simulink model "lab5_extra"  (R2017b)
settings: Solver=FixedStepDiscrete  StartTime=0.0  StopTime=5  RelTol=1e-3
InitFcn:
  | load speech_signal;
  | Fs = 8000;
  | Ts = 1/Fs;
  | 
  | DPRAM1_size = 2048; %number of words
  | DPRAM1_address_size = log2(DPRAM1_size);
  | 
  | FFT_size = 1024;
  | FFT_size_half = FFT_size;
  | FFT_frame_shift = 256;
  | FFT_frame_shift_Nbits = log2(FFT_frame_shift);
  | 
  | SysRate_Upsample_Factor = 32;
libraries: hdlsllib x16, simulink x5, dspxfrm3 x2, dspsigops x1
settings Model: Creator=Ross_admin  LastModifiedBy=s15z586
settings OptimizationCC: BlockReduction=off  ConditionallyExecuteInputs=off  DefaultParameterBehavior=Inlined
settings DebuggingCC: AlgebraicLoopMsg=error  SingleTaskRateTransMsg=error
settings HardwareCC: ProdBitPerPointer=32  ProdBitPerSizeT=32  ProdBitPerPtrDiffT=32  ProdLargestAtomicFloat=None  ProdIntDivRoundTo=Undefined  ProdEndianess=Unspecified  ProdWordSize=32  ProdHWDeviceType=ASIC/FPGA->ASIC/FPGA  TargetBitPerPointer=64  TargetBitPerSizeT=64  TargetBitPerPtrDiffT=64  TargetLongLongMode=on  TargetIntDivRoundTo=Zero  TargetEndianess=LittleEndian  TargetWordSize=64  TargetHWDeviceType=Custom Processor->MATLAB Host Computer  ProdEqTarget=off
settings CodeAppCC: StateflowObjectComments=on

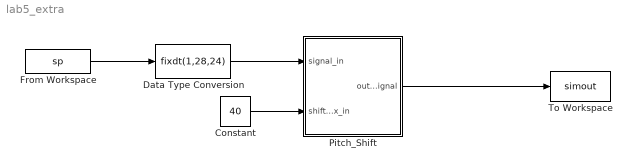
== system lab5_extra ==
  Constant : Constant  Value=40  OutDataTypeStr=fixdt(1,16,0)  SampleTime=Ts
  Data Type Conversion : DataTypeConversion  OutDataTypeStr=fixdt(1,28,24)
  From Workspace : FromWorkspace  VariableName=sp  SampleTime=Ts
  Pitch_Shift : Subsystem
  To Workspace : ToWorkspace  VariableName=simout  SampleTime=-1
  wires:
  Pitch_Shift/1(output_signal) -> To Workspace/1
  Constant/1 -> Pitch_Shift/2(shift_index_in)
  Data Type Conversion/1 -> Pitch_Shift/1(signal_in)
  From Workspace/1 -> Data Type Conversion/1

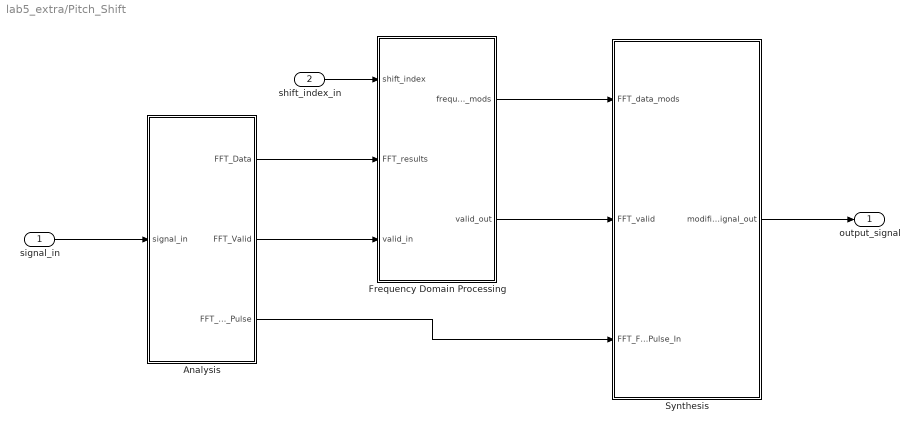
== system lab5_extra/Pitch_Shift ==
  signal_in : Inport
  shift_index_in : Inport  Port=2
  Analysis : Subsystem
  Frequency Domain Processing : Subsystem
  Synthesis : Subsystem
  output_signal : Outport
  wires:
  signal_in/1 -> Analysis/1(signal_in)
  Synthesis/1(modified_signal_out) -> output_signal/1
  Frequency Domain Processing/2(valid_out) -> Synthesis/2(FFT_valid)
  Analysis/3(FFT_Frame_Pulse) -> Synthesis/3(FFT_Frame_Pulse_In)
  Analysis/1(FFT_Data) -> Frequency Domain Processing/2(FFT_results)
  Analysis/2(FFT_Valid) -> Frequency Domain Processing/3(valid_in)
  Frequency Domain Processing/1(frequency_mods) -> Synthesis/1(FFT_data_mods)
  shift_index_in/1 -> Frequency Domain Processing/1(shift_index)

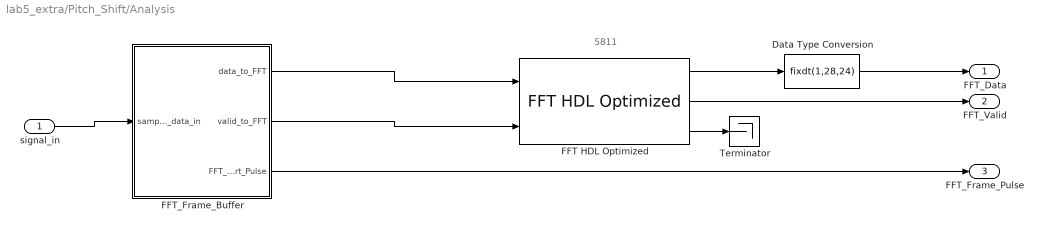
== system lab5_extra/Pitch_Shift/Analysis ==
  note: 5811
  signal_in : Inport
  Data Type Conversion : DataTypeConversion  OutDataTypeStr=fixdt(1,28,24)
  FFT HDL Optimized : dspxfrm3/FFT HDL Optimized  FFTLength=1024  Architecture=Burst Radix 2  ComplexMultiplication=Use 4 multipliers and 2 adders  BitReversedOutput=off  BitReversedInput=off  Normalize=on  SimulateUsing=Code generation  RoundingMethod=Floor  ResetInputPort=off  StartOutputPort=off  EndOutputPort=off
      settings: SourceProductName=DSP System Toolbox  SourceProductBaseCode=DS
  FFT_Frame_Buffer : Subsystem
  Terminator : Terminator
  FFT_Data : Outport
  FFT_Valid : Outport  Port=2
  FFT_Frame_Pulse : Outport  Port=3
  wires:
  signal_in/1 -> FFT_Frame_Buffer/1(sample_data_in)
  FFT_Frame_Buffer/1(data_to_FFT) -> FFT HDL Optimized/1
  FFT HDL Optimized/2 -> FFT_Valid/1
  FFT_Frame_Buffer/3(FFT_Frame_Start_Pulse) -> FFT_Frame_Pulse/1
  FFT HDL Optimized/3 -> Terminator/1
  FFT HDL Optimized/1 -> Data Type Conversion/1
  Data Type Conversion/1 -> FFT_Data/1
  FFT_Frame_Buffer/2(valid_to_FFT) -> FFT HDL Optimized/2

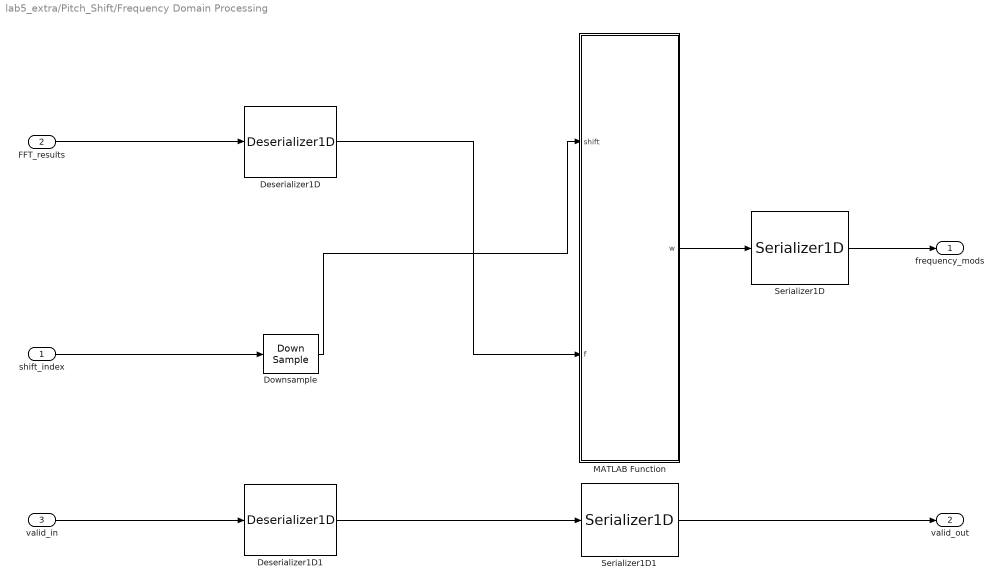
== system lab5_extra/Pitch_Shift/Frequency Domain Processing ==
  shift_index : Inport
  FFT_results : Inport  Port=2
  valid_in : Inport  Port=3
  Deserializer1D : hdlsllib/HDL Operations/Deserializer1D  Ratio=1024  IdleCycles=0  InitialCondition=0  startIn=off  validIn=off  validOut=off  inputDataDimensions=-1  inputSampleTime=-1  inputSignalType=auto
      settings: SourceProductName=HDL Coder  SourceProductBaseCode=HD
  Deserializer1D1 : hdlsllib/HDL Operations/Deserializer1D  Ratio=1024  IdleCycles=0  InitialCondition=0  startIn=off  validIn=off  validOut=off  inputDataDimensions=-1  inputSampleTime=-1  inputSignalType=auto
      settings: SourceProductName=HDL Coder  SourceProductBaseCode=HD
  Downsample : DownSample  N=FFT_size/SysRate_Upsample_Factor  RateOptions=Allow multirate processing
  MATLAB Function : MATLAB Function  TreatAsAtomicUnit=on
  Serializer1D : hdlsllib/HDL Operations/Serializer1D  Ratio=1024  IdleCycles=0  validIn=off  startOut=off  validOut=off  inputDataDimensions=-1  inputSampleTime=-1  inputSignalType=auto
      settings: SourceProductName=HDL Coder  SourceProductBaseCode=HD
  Serializer1D1 : hdlsllib/HDL Operations/Serializer1D  Ratio=1024  IdleCycles=0  validIn=off  startOut=off  validOut=off  inputDataDimensions=-1  inputSampleTime=-1  inputSignalType=auto
      settings: SourceProductName=HDL Coder  SourceProductBaseCode=HD
  frequency_mods : Outport
  valid_out : Outport  Port=2
  wires:
  shift_index/1 -> Downsample/1
  FFT_results/1 -> Deserializer1D/1
  valid_in/1 -> Deserializer1D1/1
  Deserializer1D1/1 -> Serializer1D1/1
  MATLAB Function/1(w) -> Serializer1D/1
  Serializer1D/1 -> frequency_mods/1
  Serializer1D1/1 -> valid_out/1
  Downsample/1 -> MATLAB Function/1(shift)
  Deserializer1D/1 -> MATLAB Function/2(f)

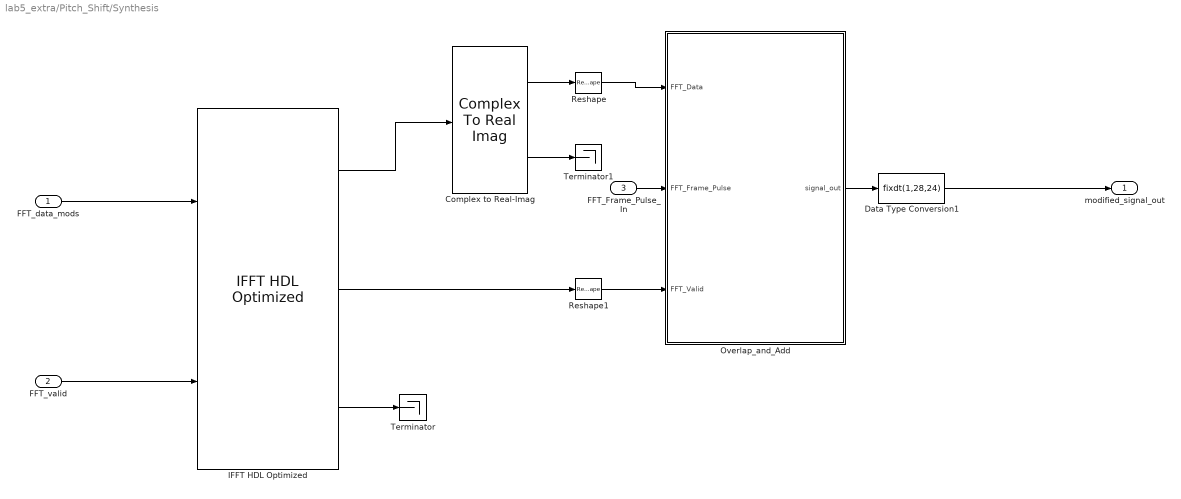
== system lab5_extra/Pitch_Shift/Synthesis ==
  FFT_data_mods : Inport
  FFT_valid : Inport  Port=2
  FFT_Frame_Pulse_In : Inport  Port=3
  Complex to Real-Imag : ComplexToRealImag
  Data Type Conversion1 : DataTypeConversion  OutDataTypeStr=fixdt(1,28,24)
  IFFT HDL Optimized : dspxfrm3/IFFT HDL Optimized  FFTLength=1024  Architecture=Burst Radix 2  ComplexMultiplication=Use 4 multipliers and 2 adders  BitReversedOutput=off  BitReversedInput=off  Normalize=on  SimulateUsing=Code generation  RoundingMethod=Floor  ResetInputPort=off  StartOutputPort=off  EndOutputPort=off
      settings: SourceProductName=DSP System Toolbox  SourceProductBaseCode=DS
  Overlap_and_Add : Subsystem
  Reshape : Reshape
  Reshape1 : Reshape
  Terminator : Terminator
  Terminator1 : Terminator
  modified_signal_out : Outport
  wires:
  FFT_data_mods/1 -> IFFT HDL Optimized/1
  FFT_valid/1 -> IFFT HDL Optimized/2
  FFT_Frame_Pulse_In/1 -> Overlap_and_Add/2(FFT_Frame_Pulse)
  IFFT HDL Optimized/3 -> Terminator/1
  IFFT HDL Optimized/1 -> Complex to Real-Imag/1
  Complex to Real-Imag/2 -> Terminator1/1
  Complex to Real-Imag/1 -> Reshape/1
  Reshape/1 -> Overlap_and_Add/1(FFT_Data)
  IFFT HDL Optimized/2 -> Reshape1/1
  Reshape1/1 -> Overlap_and_Add/3(FFT_Valid)
  Overlap_and_Add/1(signal_out) -> Data Type Conversion1/1
  Data Type Conversion1/1 -> modified_signal_out/1

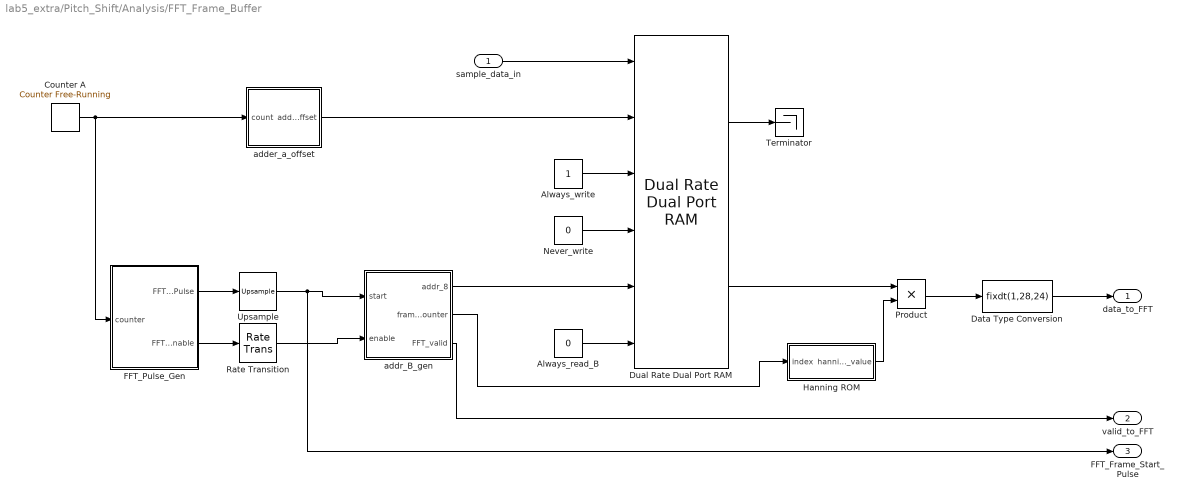
== system lab5_extra/Pitch_Shift/Analysis/FFT_Frame_Buffer ==
  sample_data_in : Inport
  Always_read_B : Constant  Value=0  OutDataTypeStr=boolean  SampleTime=Ts/SysRate_Upsample_Factor
  Always_write : Constant  OutDataTypeStr=boolean  SampleTime=Ts
  Counter A : simulink/Sources/Counter Free-Running  NumBits=DPRAM1_address_size  tsamp=Ts
  Data Type Conversion : DataTypeConversion  OutDataTypeStr=fixdt(1,28,24)
  Dual Rate Dual Port RAM : hdlsllib/HDL RAMs/Dual Rate Dual Port RAM  ram_size=DPRAM1_address_size
      settings: SourceProductName=HDL Coder  SourceProductBaseCode=HD
  FFT_Pulse_Gen : Subsystem
  Hanning ROM : Subsystem
  Never_write : Constant  Value=0  OutDataTypeStr=fixdt(1,28,24)  SampleTime=Ts/SysRate_Upsample_Factor
  Product : Product
  Rate Transition : RateTransition  OutPortSampleTimeOpt=Multiple of input port sample time  OutPortSampleTimeMultiple=1/SysRate_Upsample_Factor  OutPortSampleTime=1/SysRate_Upsample_Factor
  Terminator : Terminator
  Upsample : dspsigops/Upsample  N=SysRate_Upsample_Factor  phase=0  RateOptions=Allow multirate processing  ic=0  mode=Unused parameter value
  adder_a_offset : Subsystem
  addr_B_gen : Subsystem
  data_to_FFT : Outport
  valid_to_FFT : Outport  Port=2
  FFT_Frame_Start_Pulse : Outport  Port=3
  wires:
  sample_data_in/1 -> Dual Rate Dual Port RAM/1
  Never_write/1 -> Dual Rate Dual Port RAM/4
  Always_write/1 -> Dual Rate Dual Port RAM/3
  Always_read_B/1 -> Dual Rate Dual Port RAM/6
  Counter A/1 -> adder_a_offset/1(count), FFT_Pulse_Gen/1(counter)
  Dual Rate Dual Port RAM/1 -> Terminator/1
  Upsample/1 -> FFT_Frame_Start_Pulse/1, addr_B_gen/1(start)
  FFT_Pulse_Gen/1(FFT_Start_Pulse) -> Upsample/1
  Dual Rate Dual Port RAM/2 -> Product/1
  Product/1 -> Data Type Conversion/1
  adder_a_offset/1(addr_offset) -> Dual Rate Dual Port RAM/2
  addr_B_gen/1(addr_8) -> Dual Rate Dual Port RAM/5
  addr_B_gen/3(FFT_valid) -> valid_to_FFT/1
  Data Type Conversion/1 -> data_to_FFT/1
  addr_B_gen/2(frame_counter) -> Hanning ROM/1(index)
  Hanning ROM/1(hanning_value) -> Product/2
  FFT_Pulse_Gen/2(FFT_enable) -> Rate Transition/1
  Rate Transition/1 -> addr_B_gen/2(enable)

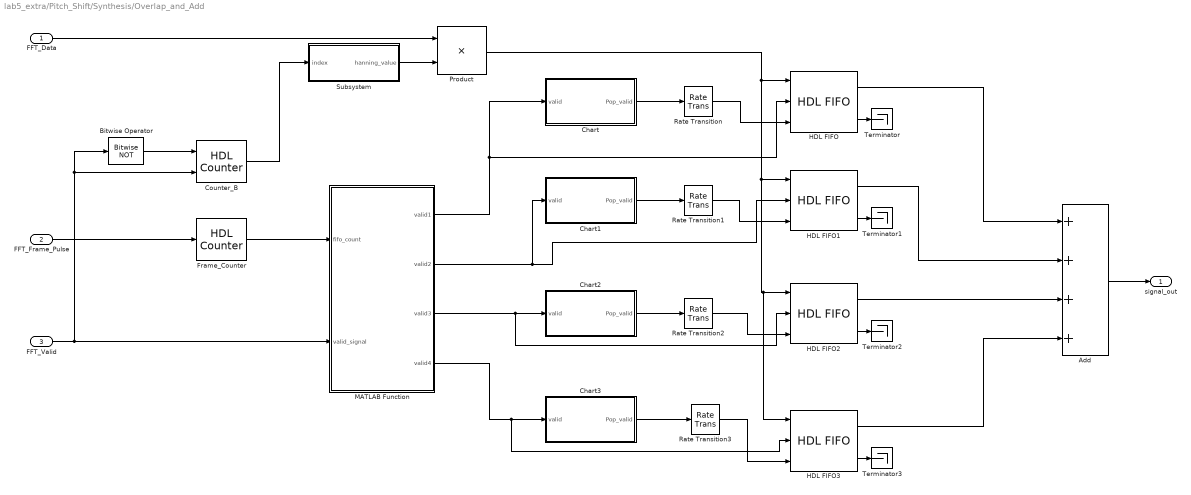
== system lab5_extra/Pitch_Shift/Synthesis/Overlap_and_Add ==
  FFT_Data : Inport
  FFT_Frame_Pulse : Inport  Port=2
  FFT_Valid : Inport  Port=3
  Add : Sum  Inputs=++++
  Bitwise Operator : simulink/Logic and Bit Operations/Bitwise Operator  logicop=NOT  UseBitMask=off  BitMask=bin2dec('11011001')  BitMaskRealWorld=Stored Integer
  Chart : Stateflow chart  TreatAsAtomicUnit=on
  Chart1 : Stateflow chart  TreatAsAtomicUnit=on
  Chart2 : Stateflow chart  TreatAsAtomicUnit=on
  Chart3 : Stateflow chart  TreatAsAtomicUnit=on
  Counter_B : hdlsllib/Sources/HDL Counter  CountType=Count limited  CountInit=0  CountStep=1  CountMax=FFT_size  CountFromType=Initial value  CountFrom=0  CountResetPort=on  CountLoadPort=off  CountEnbPort=on  CountDirPort=off  CountDataType=Unsigned  CountWordLen=DPRAM1_address_size  CountFracLen=0  CountSampTime=1
      settings: SourceProductBaseCode=HD
  Frame_Counter : hdlsllib/Sources/HDL Counter  CountType=Free running  CountInit=2  CountStep=1  CountMax=4  CountFromType=Initial value  CountFrom=2  CountResetPort=off  CountLoadPort=off  CountEnbPort=on  CountDirPort=off  CountDataType=Unsigned  CountWordLen=2  CountFracLen=0  CountSampTime=1
      settings: SourceProductBaseCode=HD
  HDL FIFO{,1..3} (4 alike) : hdlsllib/HDL RAMs/HDL FIFO  fifo_size=FFT_size  ratio=SysRate_Upsample_Factor  push_msg=Warning  pop_msg=Warning  show_empty=off  show_full=on  show_num=off
      settings: SourceProductName=HDL Coder  SourceProductBaseCode=HD
  MATLAB Function : MATLAB Function  TreatAsAtomicUnit=on
  Product : Product
  Rate Transition{,1..3} (4 alike) : RateTransition  OutPortSampleTimeOpt=Multiple of input port sample time  OutPortSampleTimeMultiple=SysRate_Upsample_Factor  OutPortSampleTime=SysRate_Upsample_Factor
  Subsystem : Subsystem
  Terminator{,1..3} (4 alike) : Terminator
  signal_out : Outport
  wires:
  FFT_Data/1 -> Product/1
  FFT_Frame_Pulse/1 -> Frame_Counter/1
  HDL FIFO1/2 -> Terminator1/1
  HDL FIFO3/2 -> Terminator3/1
  HDL FIFO2/2 -> Terminator2/1
  HDL FIFO/2 -> Terminator/1
  MATLAB Function/2(valid2) -> Chart1/1(valid), HDL FIFO1/2
  Rate Transition/1 -> HDL FIFO/3
  Rate Transition1/1 -> HDL FIFO1/3
  Rate Transition2/1 -> HDL FIFO2/3
  Rate Transition3/1 -> HDL FIFO3/3
  Product/1 -> HDL FIFO3/1, HDL FIFO2/1, HDL FIFO1/1, HDL FIFO/1
  Bitwise Operator/1 -> Counter_B/1
  Subsystem/1(hanning_value) -> Product/2
  Counter_B/1 -> Subsystem/1(index)
  Frame_Counter/1 -> MATLAB Function/1(fifo_count)
  FFT_Valid/1 -> Counter_B/2, Bitwise Operator/1, MATLAB Function/2(valid_signal)
  HDL FIFO/1 -> Add/1
  HDL FIFO1/1 -> Add/2
  HDL FIFO2/1 -> Add/3
  HDL FIFO3/1 -> Add/4
  Add/1 -> signal_out/1
  MATLAB Function/1(valid1) -> HDL FIFO/2, Chart/1(valid)
  Chart/1(Pop_valid) -> Rate Transition/1
  Chart1/1(Pop_valid) -> Rate Transition1/1
  Chart2/1(Pop_valid) -> Rate Transition2/1
  MATLAB Function/3(valid3) -> HDL FIFO2/2, Chart2/1(valid)
  Chart3/1(Pop_valid) -> Rate Transition3/1
  MATLAB Function/4(valid4) -> HDL FIFO3/2, Chart3/1(valid)

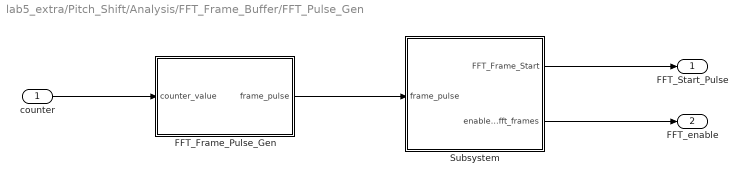
== system lab5_extra/Pitch_Shift/Analysis/FFT_Frame_Buffer/FFT_Pulse_Gen ==
  counter : Inport
  FFT_Frame_Pulse_Gen : Subsystem
  Subsystem : Subsystem
  FFT_Start_Pulse : Outport
  FFT_enable : Outport  Port=2
  wires:
  counter/1 -> FFT_Frame_Pulse_Gen/1(counter_value)
  Subsystem/1(FFT_Frame_Start) -> FFT_Start_Pulse/1
  FFT_Frame_Pulse_Gen/1(frame_pulse) -> Subsystem/1(frame_pulse)
  Subsystem/2(enable_fft_frames) -> FFT_enable/1

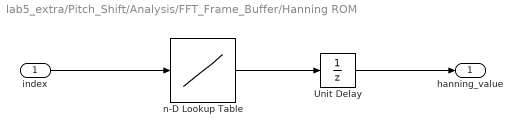
== system lab5_extra/Pitch_Shift/Analysis/FFT_Frame_Buffer/Hanning ROM ==
  index : Inport
  Unit Delay : UnitDelay  SampleTime=-1
  n-D Lookup Table : Lookup_n-D  NumberOfTableDimensions=1  LookupTableObject=''  BreakpointsForDimension1=[0:FFT_size]  BreakpointsForDimension2=[1:2]  BreakpointsForDimension3=[5, 7]  BreakpointsForDimension1FirstPoint=10  BreakpointsForDimension2FirstPoint=10  BreakpointsForDimension1Spacing=12  BreakpointsForDimension2Spacing=12  IndexSearchMethod=Evenly spaced points  Table=hanning(FFT_size+1)  InterpMethod=Flat  DiagnosticForOutOfRangeInput=Error  OutDataTypeStr=fixdt(1,16,14)  RndMeth=Simplest  InputSameDT=on
  hanning_value : Outport
  wires:
  n-D Lookup Table/1 -> Unit Delay/1
  index/1 -> n-D Lookup Table/1
  Unit Delay/1 -> hanning_value/1

== system lab5_extra/Pitch_Shift/Analysis/FFT_Frame_Buffer/adder_a_offset ==
  count : Inport
  Constant : Constant  OutDataTypeStr=fixdt(0,11,0)  SampleTime=Ts
  Sum : Sum  Inputs=|++  AccumDataTypeStr=fixdt(0,11,0)
  addr_offset : Outport
  wires:
  count/1 -> Sum/1
  Constant/1 -> Sum/2
  Sum/1 -> addr_offset/1

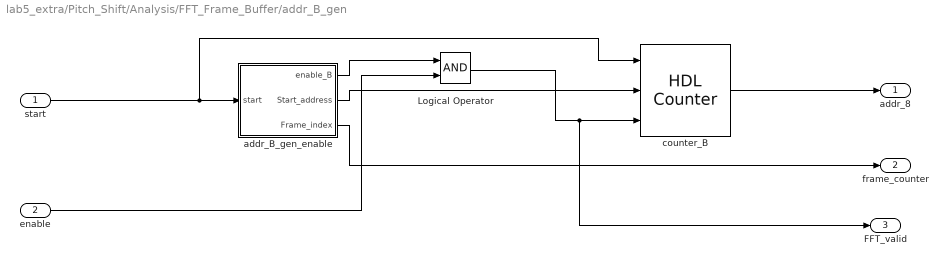
== system lab5_extra/Pitch_Shift/Analysis/FFT_Frame_Buffer/addr_B_gen ==
  start : Inport
  enable : Inport  Port=2
  Logical Operator : Logic  AllPortsSameDT=off  OutDataTypeStr=boolean
  addr_B_gen_enable : Subsystem
  counter_B : hdlsllib/Sources/HDL Counter  CountType=Free running  CountInit=DPRAM1_size-10  CountStep=1  CountMax=1024  CountFromType=Specify  CountFrom=0  CountResetPort=off  CountLoadPort=on  CountEnbPort=on  CountDirPort=off  CountDataType=Unsigned  CountWordLen=DPRAM1_address_size  CountFracLen=0  CountSampTime=1
      settings: SourceProductBaseCode=HD
  addr_8 : Outport
  frame_counter : Outport  Port=2
  FFT_valid : Outport  Port=3
  wires:
  enable/1 -> Logical Operator/2
  start/1 -> counter_B/1, addr_B_gen_enable/1(start)
  addr_B_gen_enable/1(enable_B) -> Logical Operator/1
  Logical Operator/1 -> counter_B/3, FFT_valid/1
  addr_B_gen_enable/2(Start_address) -> counter_B/2
  addr_B_gen_enable/3(Frame_index) -> frame_counter/1
  counter_B/1 -> addr_8/1

== system lab5_extra/Pitch_Shift/Synthesis/Overlap_and_Add/Subsystem ==
  index : Inport
  Unit Delay : UnitDelay  SampleTime=-1
  n-D Lookup Table : Lookup_n-D  NumberOfTableDimensions=1  LookupTableObject=''  BreakpointsForDimension1=[0:FFT_size]  BreakpointsForDimension2=[1:2]  BreakpointsForDimension3=[5, 7]  BreakpointsForDimension1FirstPoint=10  BreakpointsForDimension2FirstPoint=10  BreakpointsForDimension1Spacing=12  BreakpointsForDimension2Spacing=12  IndexSearchMethod=Evenly spaced points  Table=hanning(FFT_size+1)  InterpMethod=Flat  DiagnosticForOutOfRangeInput=Error  OutDataTypeStr=fixdt(1,16,14)  RndMeth=Simplest  InputSameDT=on
  hanning_value : Outport
  wires:
  index/1 -> n-D Lookup Table/1
  n-D Lookup Table/1 -> Unit Delay/1
  Unit Delay/1 -> hanning_value/1

== system lab5_extra/Pitch_Shift/Analysis/FFT_Frame_Buffer/FFT_Pulse_Gen/FFT_Frame_Pulse_Gen ==
  counter_value : Inport
  Bit Slice : hdlsllib/Logic and Bit Operations/Bit Slice  lidx=7  ridx=0
  Compare To Zero : simulink/Logic and Bit Operations/Compare To Zero  relop===  OutDataTypeStr=boolean
  frame_pulse : Outport
  wires:
  counter_value/1 -> Bit Slice/1
  Bit Slice/1 -> Compare To Zero/1
  Compare To Zero/1 -> frame_pulse/1

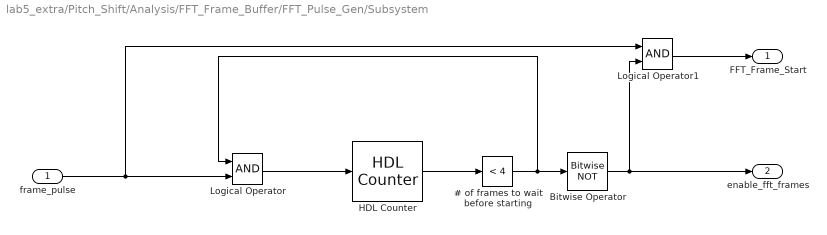
== system lab5_extra/Pitch_Shift/Analysis/FFT_Frame_Buffer/FFT_Pulse_Gen/Subsystem ==
  frame_pulse : Inport
  # of frames to wait before starting : simulink/Logic and Bit Operations/Compare To Constant  relop=<  const=4  OutDataTypeStr=boolean
  Bitwise Operator : simulink/Logic and Bit Operations/Bitwise Operator  logicop=NOT  UseBitMask=off  BitMask=bin2dec('11011001')  BitMaskRealWorld=Stored Integer
  HDL Counter : hdlsllib/Sources/HDL Counter  CountType=Count limited  CountInit=0  CountStep=1  CountMax=4  CountFromType=Specify  CountFrom=0  CountResetPort=off  CountLoadPort=off  CountEnbPort=on  CountDirPort=off  CountDataType=Unsigned  CountWordLen=5  CountFracLen=0  CountSampTime=1
      settings: SourceProductBaseCode=HD
  Logical Operator : Logic  AllPortsSameDT=off  OutDataTypeStr=boolean
  Logical Operator1 : Logic  AllPortsSameDT=off  OutDataTypeStr=boolean
  FFT_Frame_Start : Outport
  enable_fft_frames : Outport  Port=2
  wires:
  frame_pulse/1 -> Logical Operator1/1, Logical Operator/2
  Logical Operator/1 -> HDL Counter/1
  HDL Counter/1 -> # of frames to wait before starting/1
  Bitwise Operator/1 -> Logical Operator1/2, enable_fft_frames/1
  # of frames to wait before starting/1 -> Logical Operator/1, Bitwise Operator/1
  Logical Operator1/1 -> FFT_Frame_Start/1

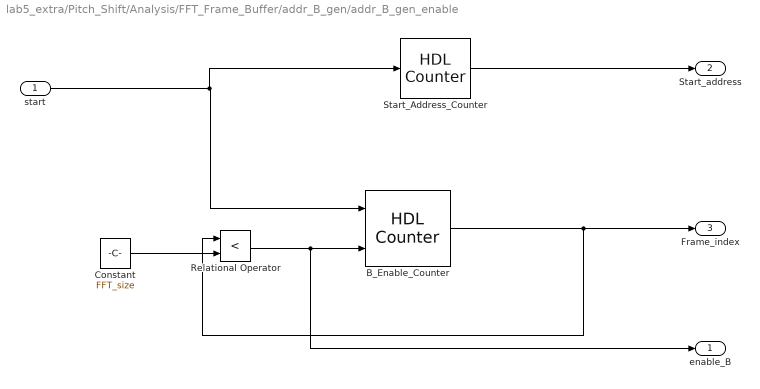
== system lab5_extra/Pitch_Shift/Analysis/FFT_Frame_Buffer/addr_B_gen/addr_B_gen_enable ==
  start : Inport
  B_Enable_Counter : hdlsllib/Sources/HDL Counter  CountType=Count limited  CountInit=0  CountStep=1  CountMax=FFT_size  CountFromType=Specify  CountFrom=0  CountResetPort=on  CountLoadPort=off  CountEnbPort=on  CountDirPort=off  CountDataType=Unsigned  CountWordLen=DPRAM1_address_size  CountFracLen=0  CountSampTime=1
      settings: SourceProductBaseCode=HD
  Constant : Constant  Value=FFT_size  OutDataTypeStr=fixdt(0,11,0)  SampleTime=Ts/SysRate_Upsample_Factor
  Relational Operator : RelationalOperator  Operator=<  OutDataTypeStr=boolean  RndMeth=Nearest
  Start_Address_Counter : hdlsllib/Sources/HDL Counter  CountType=Free running  CountInit=0  CountStep=FFT_frame_shift  CountMax=25  CountFromType=Specify  CountFrom=0  CountResetPort=off  CountLoadPort=off  CountEnbPort=on  CountDirPort=off  CountDataType=Unsigned  CountWordLen=DPRAM1_address_size  CountFracLen=0  CountSampTime=1
      settings: SourceProductBaseCode=HD
  enable_B : Outport
  Start_address : Outport  Port=2
  Frame_index : Outport  Port=3
  wires:
  start/1 -> B_Enable_Counter/1, Start_Address_Counter/1
  Relational Operator/1 -> B_Enable_Counter/2, enable_B/1
  Constant/1 -> Relational Operator/2
  B_Enable_Counter/1 -> Relational Operator/1, Frame_index/1
  Start_Address_Counter/1 -> Start_address/1

== stateflow chart lab5_extra/Pitch_Shift/Synthesis/Overlap_and_Add/Chart1 ==
  settings: executeAtInitialization=1
  state Valid_high
    entry: Pop_valid = fi(0,0,1,0);
  state Pop_assert
    entry: Pop_valid = fi(1,0,1,0);
  state Start_up
    entry: Pop_valid = fi(0,0,1,0);
  state Valid_low
    entry: Pop_valid = fi(0,0,1,0);
  (default) -> Start_up
  Valid_high -> Pop_assert [order 1] : [valid == 0]
  Start_up -> Valid_low : [valid == 0]
  Valid_low -> Valid_high [order 2] : [valid == 1]
  Valid_low -> Valid_low [order 1] : [valid == 0]
  Valid_high -> Valid_high [order 2] : [valid == 1]
  data: valid input; Pop_valid output

== matlab function lab5_extra/Pitch_Shift/Frequency Domain Processing/MATLAB Function ==
  data: shift input; f input; w output
function w = fcn(shift,f)

N = length(f);
Nd2 = N/2;
w = fi(complex(zeros(N,1)), 1, 28, 24);

if shift == 0
    w = f;
else
    w(1)     = fi(complex(0), 1 , 28, 24);
    w(Nd2+1) = fi(complex(0), 1 , 28, 24);
    
    if shift > 0  % increase the frequencies
        for i=2:Nd2
            if i <= shift
                w(i) = fi(complex(0), 1 , 28, 24); % fill in vacated positive frequencies with zeros
            else
                w(i) = f(i-shift);
            end
        end
        for i=N:-1:Nd2+2
            if i > N-shift
                w(i) = fi(complex(0), 1 , 28, 24);
            else
                w(i) = f(i+shift);
            end
        end
    end
    
    if shift < 0  % decrease the frequencies
        
        for i=Nd2:-1:2
            if i > Nd2 - shift
                w(i) = fi(complex(0), 1 , 28, 24);
            else
                w(i) = f(i-shift);
            end
        end
        
        for i=Nd2+2:N
            if i <= Nd2 +2+ shift
                w(i) = fi(complex(0), 1 , 28, 24);
            else
                w(i) = f(i+shift);
            end
        end
    end
end
end

== stateflow chart lab5_extra/Pitch_Shift/Synthesis/Overlap_and_Add/Chart ==
  settings: executeAtInitialization=1
  state Valid_high
    entry: Pop_valid = fi(0,0,1,0);
  state Pop_assert
    entry: Pop_valid = fi(1,0,1,0);
  state Start_up
    entry: Pop_valid = fi(0,0,1,0);
  state Valid_low
    entry: Pop_valid = fi(0,0,1,0);
  (default) -> Start_up
  Valid_high -> Pop_assert [order 1] : [valid == 0]
  Start_up -> Valid_low : [valid == 0]
  Valid_low -> Valid_high [order 2] : [valid == 1]
  Valid_low -> Valid_low [order 1] : [valid == 0]
  Valid_high -> Valid_high [order 2] : [valid == 1]
  data: valid input; Pop_valid output

== stateflow chart lab5_extra/Pitch_Shift/Synthesis/Overlap_and_Add/Chart2 ==
  settings: executeAtInitialization=1
  state Valid_high
    entry: Pop_valid = fi(0,0,1,0);
  state Pop_assert
    entry: Pop_valid = fi(1,0,1,0);
  state Start_up
    entry: Pop_valid = fi(0,0,1,0);
  state Valid_low
    entry: Pop_valid = fi(0,0,1,0);
  (default) -> Start_up
  Valid_high -> Pop_assert [order 1] : [valid == 0]
  Start_up -> Valid_low : [valid == 0]
  Valid_low -> Valid_high [order 2] : [valid == 1]
  Valid_low -> Valid_low [order 1] : [valid == 0]
  Valid_high -> Valid_high [order 2] : [valid == 1]
  data: valid input; Pop_valid output

== stateflow chart lab5_extra/Pitch_Shift/Synthesis/Overlap_and_Add/Chart3 ==
  settings: executeAtInitialization=1
  state Valid_high
    entry: Pop_valid = fi(0,0,1,0);
  state Pop_assert
    entry: Pop_valid = fi(1,0,1,0);
  state Start_up
    entry: Pop_valid = fi(0,0,1,0);
  state Valid_low
    entry: Pop_valid = fi(0,0,1,0);
  (default) -> Start_up
  Valid_high -> Pop_assert [order 1] : [valid == 0]
  Start_up -> Valid_low : [valid == 0]
  Valid_low -> Valid_high [order 2] : [valid == 1]
  Valid_low -> Valid_low [order 1] : [valid == 0]
  Valid_high -> Valid_high [order 2] : [valid == 1]
  data: valid input; Pop_valid output

== matlab function lab5_extra/Pitch_Shift/Synthesis/Overlap_and_Add/MATLAB Function ==
  data: fifo_count input; valid1 output; valid2 output; valid3 output; valid4 output; valid_signal input
function [valid1,valid2,valid3,valid4] = fcn(fifo_count,valid_signal)
switch(fifo_count)
    case 0
        valid1 = valid_signal;
        valid2 = false;
        valid3 = false;
        valid4 = false;
    case 1
        valid1 = false;
        valid2 = valid_signal;
        valid3 = false;
        valid4 = false;
    case 2
        valid1 = false;
        valid2 = false;
        valid3 = valid_signal;
        valid4 = false;
    case 3
        valid1 = false;
        valid2 = false;
        valid3 = false;
        valid4 = valid_signal;
    otherwise
        valid1 = false;
        valid2 = false;
        valid3 = false;
        valid4 = false;
end
